simulink model "Spring_mass_sim"  (R2020b)
settings: Solver=VariableStepAuto  StartTime=0.0  StopTime=10.0  RelTol=1e-3
values from neighbouring files (symbols this model uses):
  b = 0.1    [Spring_mass.m]
  k = 10    [Spring_mass.m]
  m = 100    [Spring_mass.m]
settings Model: Creator=isido  LastModifiedBy=isido

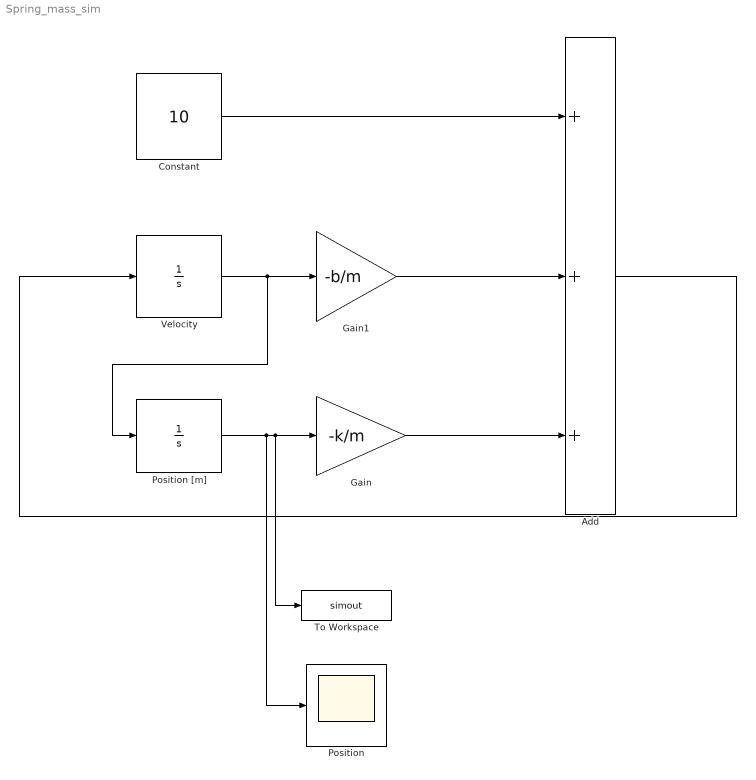
== system Spring_mass_sim ==
  Add : Sum  Inputs=+++
  Constant : Constant  Value=10
  Gain : Gain  Gain=-k/m
  Gain1 : Gain  Gain=-b/m
  Position : Scope
  Position [m] : Integrator  InitialCondition=5
  To Workspace : ToWorkspace  VariableName=simout  SaveFormat=Timeseries  SampleTime=-1
  Velocity : Integrator  InitialCondition=3
  wires:
  Position [m]/1 -> Position/1, To Workspace/1, Gain/1
  Velocity/1 -> Position [m]/1, Gain1/1
  Constant/1 -> Add/1
  Gain1/1 -> Add/2
  Gain/1 -> Add/3
  Add/1 -> Velocity/1
